simulink model "CAR_CONTROL_SYSTEM"  (R2024b)
settings: Solver=FixedStepAuto  StartTime=0.0  StopTime=inf  FixedStep=1e-3  RelTol=1e-3  EnableMultiTasking=on
model workspace (MAT data in the model file):
  SL_ROS_VariableLengthArrays_MaxSizes : object (value not decoded)
undefined symbols (not defined in the file or in its folder): angular, CIRCUIT, CLTF_DAMP, CLTF_FREQ, CLTF_GAIN, CONTROL, CONTROL_INI, DiscIntNeverNeededParam, dspblkCoreblockFVToolHelper, gcbh, INPUT, linear, MCP3201, MD25, MODEL, MODEL_INI, mpcstate, MPU60X0, MPU9250, MSG, NAV_MPC_CONTROL, OUTPUT, SAMPLING_TIME, SYSID_INPUT, VL6180X
libraries: raspberrypiCommlib x153, simulink x85, raspberrypiNetworklib x8, embedlinuxBasiclib x6, ctrlSharedLib x2, ros2lib x2, mpclib x1, vrlib x1, sldrtlib x1
(part 9 of 16)

== system CAR_CONTROL_SYSTEM/HARDWARE/SENSORS/WALL RANGE SENSOR/VL6180X_I2C_FRONT/VL6180X INITIALIZATION/MEASUREMENT CONFIGURATION/START READ RANGE SINGLE/I2C WRITE: SYSRANGE_START ==
  DATA : Inport
  Constant : Constant  Value=REGISTER_ADDRESS_MSB  OutDataTypeStr=uint8  SampleTime=SAMPLING_TIME
  Constant1 : Constant  Value=REGISTER_ADDRESS_LSB  OutDataTypeStr=uint8  SampleTime=SAMPLING_TIME
  Mux : Mux  Inputs=3
  REGISTER ADDRESS : raspberrypiCommlib/I2C Controller Write  Priority=10  BoardProperty=Pi 3 Model B+  I2CModule=1  Mode=Master  SlaveAddress=SLAVE_ADDRESS  SlaveByteOrder=BigEndian  Direction=Transmitter  RegisterAddressMode=off  RegisterAddress=hex2dec('207')  SlaveDataType=uint8  DataLength=1  NoAck=off  RepeatedStart=off  OutputStatus=off
  wires:
  Mux/1 -> REGISTER ADDRESS/1
  Constant/1 -> Mux/1
  DATA/1 -> Mux/3
  Constant1/1 -> Mux/2

== system CAR_CONTROL_SYSTEM/HARDWARE/SENSORS/WALL RANGE SENSOR/VL6180X_I2C_REAR/VL6180X INITIALIZATION/MEASUREMENT CONFIGURATION/START READ RANGE CONTINUOUS/I2C WRITE: SYSRANGE_START ==
  DATA : Inport
  Constant : Constant  Value=REGISTER_ADDRESS_MSB  OutDataTypeStr=uint8  SampleTime=SAMPLING_TIME
  Constant1 : Constant  Value=REGISTER_ADDRESS_LSB  OutDataTypeStr=uint8  SampleTime=SAMPLING_TIME
  Mux : Mux  Inputs=3
  REGISTER ADDRESS : raspberrypiCommlib/I2C Controller Write  Priority=10  BoardProperty=Pi 3 Model B+  I2CModule=1  Mode=Master  SlaveAddress=SLAVE_ADDRESS  SlaveByteOrder=BigEndian  Direction=Transmitter  RegisterAddressMode=off  RegisterAddress=hex2dec('207')  SlaveDataType=uint8  DataLength=1  NoAck=off  RepeatedStart=off  OutputStatus=off
  wires:
  Constant1/1 -> Mux/2
  DATA/1 -> Mux/3
  Constant/1 -> Mux/1
  Mux/1 -> REGISTER ADDRESS/1

== system CAR_CONTROL_SYSTEM/HARDWARE/SENSORS/WALL RANGE SENSOR/VL6180X_I2C_REAR/VL6180X INITIALIZATION/MEASUREMENT CONFIGURATION/START READ RANGE SINGLE/I2C WRITE: SYSRANGE_START ==
  DATA : Inport
  Constant : Constant  Value=REGISTER_ADDRESS_MSB  OutDataTypeStr=uint8  SampleTime=SAMPLING_TIME
  Constant1 : Constant  Value=REGISTER_ADDRESS_LSB  OutDataTypeStr=uint8  SampleTime=SAMPLING_TIME
  Mux : Mux  Inputs=3
  REGISTER ADDRESS : raspberrypiCommlib/I2C Controller Write  Priority=10  BoardProperty=Pi 3 Model B+  I2CModule=1  Mode=Master  SlaveAddress=SLAVE_ADDRESS  SlaveByteOrder=BigEndian  Direction=Transmitter  RegisterAddressMode=off  RegisterAddress=hex2dec('207')  SlaveDataType=uint8  DataLength=1  NoAck=off  RepeatedStart=off  OutputStatus=off
  wires:
  Constant1/1 -> Mux/2
  DATA/1 -> Mux/3
  Constant/1 -> Mux/1
  Mux/1 -> REGISTER ADDRESS/1

== matlab function CAR_CONTROL_SYSTEM/SIMULATION/SENSOR MODEL ==
  data: MODEL input; CONTROL_IN input; CONTROL output Bus: CONTROL_Bus; SENSOR_NOISE input
function CONTROL = SENSOR_MODEL(MODEL,CONTROL_IN,SENSOR_NOISE)

%--------------------------------------------------------------
% COPY CONTROL BUS
%--------------------------------------------------------------
CONTROL = CONTROL_IN;

%--------------------------------------------------------------
% STATE
%--------------------------------------------------------------
persistent initialize LIDAR_2D_ANG

if isempty(initialize)
    LIDAR_2D_ANG = 30;
    initialize = 1;
end

%--------------------------------------------------------------
% SENSOR PARAMETERS
%--------------------------------------------------------------
% Range sensor distance (m)
d_sens = MODEL.PARAM.RANGE_SENS_DIST;
% Standard deviation for range sensor (m)
RANGE_DIST_NOISE = MODEL.PARAM.RANGE_DIST_NOISE;
% Distance between range sensors (m)
RANGE_SENS_DIST = MODEL.PARAM.RANGE_SENS_DIST;
% Standard deviation for Lidar 2D (m and rad)
LIDAR_2D_DIST_NOISE = MODEL.PARAM.LIDAR_2D_DIST_NOISE;
LIDAR_2D_ANG_NOISE = MODEL.PARAM.LIDAR_2D_ANG_NOISE;

%--------------------------------------------------------------
% MODEL OUTPUT READ
%--------------------------------------------------------------
WALL_DIST = MODEL.OUTPUT.WALL_DIST;
WALL_ANG = MODEL.OUTPUT.WALL_ANG;

%--------------------------------------------------------------
% LIDAR 2D READOUT
%--------------------------------------------------------------
if CONTROL.STATE.WALL_FOLLOWER_MODE % LIDAR 2D
    % LIDAR ROTATION 360 deg/80 ms
    aux1 = LIDAR_2D_ANG + 45*sort(rand(20,1));
    aux1 =  rem(aux1,360);
    LIDAR_2D_ANG = aux1(end);
    % The Lidar 2D 0 deg axis coincides with the vehicle negative X axis
    % The Lidar 2D rotates clockwise
    aux2 = CONTROL.EKF_WFL.PARAM.LIDAR_2D_WFL_ANG_SIGN*aux1 + ...
        CONTROL.EKF_WFL.PARAM.LIDAR_2D_WFL_ANG_OFFS;
    LIDAR_2D_WALL_DIST = -ones(120,1);
    LIDAR_2D_WALL_ANG = -ones(120,1);
    ind = aux2>=-45 & aux2<=45;
    if sum(ind)>0
        LIDAR_2D_WALL_DIST(ind) = WALL_DIST./cosd(aux2(ind)-180/pi*WALL_ANG) + ...
            LIDAR_2D_DIST_NOISE*randn(sum(ind),1)*double(MODEL.PARAM.NOISE_FLAG);
        LIDAR_2D_WALL_ANG(ind) = aux1(ind) + ...
            180/pi*LIDAR_2D_ANG_NOISE*randn(sum(ind),1)*double(MODEL.PARAM.NOISE_FLAG);
    end
    % [ANGLE(deg) DISTANCE(m)]: up to 20 measurements available each sampling time
    CONTROL.INPUT.LIDAR_2D = [LIDAR_2D_WALL_ANG LIDAR_2D_WALL_DIST];
else % RANGE SENSOR
    %  d_front + d_rear = 2*d_wall/cos(Shi_wall)
    % -d_front + d_rear = d_sens*tan(Shi_wall)
    aux = [1 1 ; -1 1]\[2*WALL_DIST/cos(WALL_ANG) ; d_sens*tan(WALL_ANG)];
    FRONT_DIST = aux(1);
    REAR_DIST = aux(2);
    RANGE_FRONT_DIST = FRONT_DIST + SENSOR_NOISE(1)*RANGE_DIST_NOISE;
    RANGE_REAR_DIST = REAR_DIST + SENSOR_NOISE(2)*RANGE_DIST_NOISE;
    RANGE_WALL_ANG = atan2(RANGE_REAR_DIST-RANGE_FRONT_DIST,RANGE_SENS_DIST);
    RANGE_WALL_DIST = (RANGE_FRONT_DIST+RANGE_REAR_DIST)/2*cos(RANGE_WALL_ANG);
    CONTROL.INPUT.RANGE_FRONT_DIST = RANGE_FRONT_DIST; % m
    CONTROL.INPUT.RANGE_REAR_DIST = RANGE_REAR_DIST; % m
    CONTROL.INPUT.RANGE_WALL_ANG = RANGE_WALL_ANG; % m
    CONTROL.INPUT.RANGE_WALL_DIST = RANGE_WALL_DIST; % m
end

%--------------------------------------------------------------
% MOTION CAPTURE SYSTEM
%--------------------------------------------------------------
CONTROL.INPUT.MCS_EULER_ANG = MODEL.OUTPUT.EULER_ANG-CONTROL.PARAM.MCS_EULER_ANG_OFFS; % rad
CONTROL.INPUT.MCS_EARTH_POS = MODEL.OUTPUT.EARTH_POS-CONTROL.PARAM.MCS_EARTH_POS_OFFS; % m
if CONTROL.STATE.CURRENT_STATUS_SYS>1
    CONTROL.INPUT.MCS_EARTH_POS = CONTROL.INPUT.MCS_EARTH_POS - CONTROL.PARAM.MCS_EARTH_POS_OFFS;
    CONTROL.INPUT.MCS_EULER_ANG = CONTROL.INPUT.MCS_EULER_ANG - CONTROL.PARAM.MCS_EULER_ANG_OFFS;
end
% UNWRAPPING
yaw_ang = CONTROL.INPUT.MCS_EULER_ANG(3);
yaw_ang_ref = CONTROL.TARGET.YAW_ANG_REF;
angle_error = yaw_ang_ref - yaw_ang;
if abs(angle_error) > pi
    if yaw_ang <= 0
        yaw_ang = yaw_ang + 2*pi;
    else
        yaw_ang = yaw_ang - 2*pi;
    end
    CONTROL.INPUT.MCS_EULER_ANG(3) = yaw_ang;
end

%--------------------------------------------------------------
% NAVIGATION
%--------------------------------------------------------------
% NAVIGATION SYSTEM
CONTROL.INPUT.NAV_EULER_ANG = MODEL.OUTPUT.EULER_ANG-CONTROL.PARAM.NAV_EULER_ANG_OFFS; % rad
CONTROL.INPUT.NAV_EARTH_POS = MODEL.OUTPUT.EARTH_POS-CONTROL.PARAM.NAV_EARTH_POS_OFFS; % m
if CONTROL.STATE.CURRENT_STATUS_SYS>1
    CONTROL.INPUT.NAV_EARTH_POS = CONTROL.INPUT.NAV_EARTH_POS - CONTROL.PARAM.NAV_EARTH_POS_OFFS;
    CONTROL.INPUT.NAV_EULER_ANG = CONTROL.INPUT.NAV_EULER_ANG - CONTROL.PARAM.NAV_EULER_ANG_OFFS;
end
% UNWRAPPING
yaw_ang = CONTROL.INPUT.NAV_EULER_ANG(3);
yaw_ang_ref = CONTROL.TARGET.YAW_ANG_REF;
angle_error = yaw_ang_ref - yaw_ang;
if abs(angle_error) > pi
    if yaw_ang <= 0
        yaw_ang = yaw_ang + 2*pi;
    else
        yaw_ang = yaw_ang - 2*pi;
    end
    CONTROL.INPUT.NAV_EULER_ANG(3) = yaw_ang;
end

return
